simulink subsystem "Sub_Encoders"  (R2023b)
settings: Solver=VariableStepAuto  StartTime=0.0  StopTime=10.0  RelTol=1e-3
libraries: arduinosensorlib x2, simulink x1
settings Model: Creator=Usuario  LastModifiedBy=Usuario

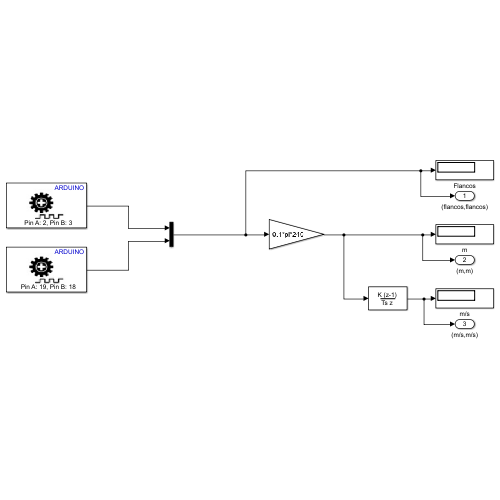
[thumbnail: Simulink's stored preview of the top-level diagram]
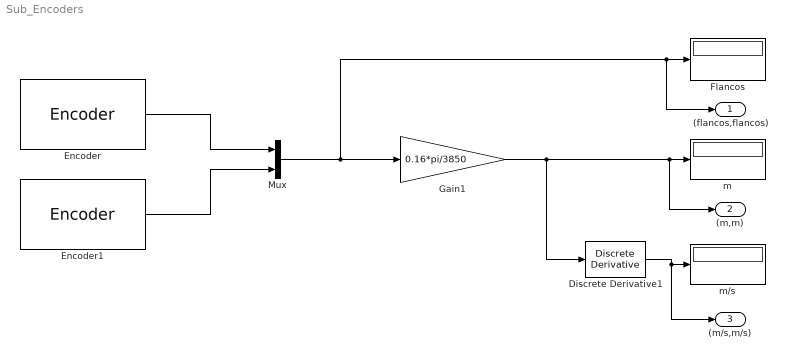
== system Sub_Encoders ==
  Discrete Derivative1 : simulink/Discrete/Discrete Derivative  gainval=1.0  ICPrevScaledInput=0.0  OutMin=[]  OutMax=[]  OutDataType=fixdt(1, 16)  OutScaling=2^-10  DoSatur=off
  Encoder : arduinosensorlib/Encoder  InputA=2  InputB=3  Mode=No reset  SampleTime=-1
  Encoder1 : arduinosensorlib/Encoder  InputA=18  InputB=19  Mode=No reset  SampleTime=-1
  Flancos : Display
  Gain1 : Gain  Gain=0.16*pi/3850
  Mux : Mux  Inputs=2
  m : Display
  m/s : Display
  (flancos,flancos) : Outport
  (m,m) : Outport  Port=2
  (m/s,m/s) : Outport  Port=3
  wires:
  Gain1/1 -> Discrete Derivative1/1, m/1, (m,m)/1
  Discrete Derivative1/1 -> (m/s,m/s)/1, m/s/1
  Mux/1 -> Flancos/1, (flancos,flancos)/1, Gain1/1
  Encoder/1 -> Mux/1
  Encoder1/1 -> Mux/2
